simulink model "set_point_discreto"  (R2023b)
settings: Solver=VariableStepAuto  StartTime=0.0  StopTime=10.0  RelTol=1e-3
values from neighbouring files (symbols this model uses):
  r = 120.0    (= 120)    [controlador_foc_simulink.m]    (also in parametros_planta.m; params_subsistema_mecanico.m; sistema_completo_en_codigo.m)
  Ts = interp_ts(Ts_ts,t)    [calcular_metricas_operacion.m]
settings Model: Creator=Pc  LastModifiedBy=Pc

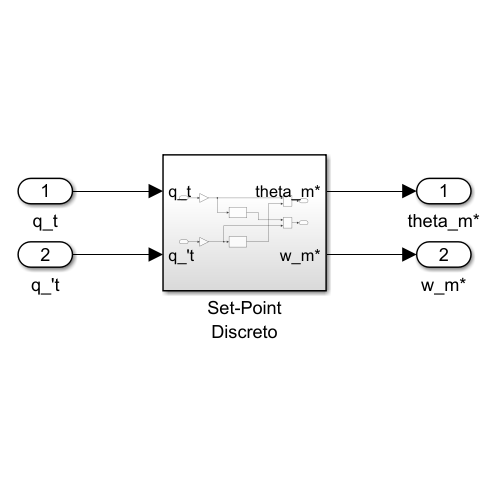
[thumbnail: Simulink's stored preview of the top-level diagram]
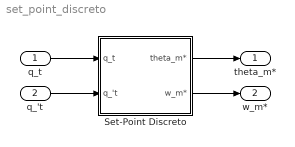
== system set_point_discreto ==
  q_t : Inport
  q_'t : Inport  Port=2
  Set-Point Discreto : Subsystem
  theta_m* : Outport
  w_m* : Outport  Port=2
  wires:
  Set-Point Discreto/1(theta_m*) -> theta_m*/1
  Set-Point Discreto/2(w_m*) -> w_m*/1
  q_t/1 -> Set-Point Discreto/1(q_t)
  q_'t/1 -> Set-Point Discreto/2(q_'t)

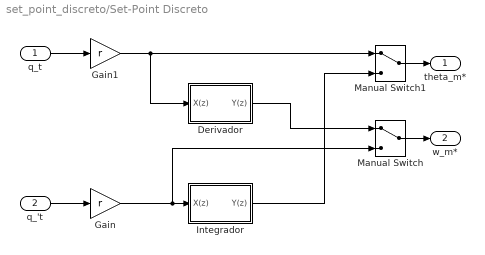
== system set_point_discreto/Set-Point Discreto ==
  q_t : Inport
  q_'t : Inport  Port=2
  "Derivador " : Subsystem
  Gain : Gain  Gain=r
  Gain1 : Gain  Gain=r
  Integrador : Subsystem
  Manual Switch : ManualSwitch
  Manual Switch1 : ManualSwitch
  theta_m* : Outport
  w_m* : Outport  Port=2
  wires:
  "Derivador "/1(Y(z)) -> Manual Switch/1
  Manual Switch/1 -> w_m*/1
  q_t/1 -> Gain1/1
  Gain1/1 -> "Derivador "/1(X(z)), Manual Switch1/1
  q_'t/1 -> Gain/1
  Manual Switch1/1 -> theta_m*/1
  Gain/1 -> Manual Switch/2, Integrador/1(X(z))
  Integrador/1(Y(z)) -> Manual Switch1/2

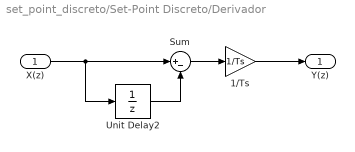
== system set_point_discreto/Set-Point Discreto/Derivador  ==
  X(z) : Inport
  1/Ts : Gain  Gain=1/Ts
  Sum : Sum  Inputs=|+-
  Unit Delay2 : UnitDelay  SampleTime=Ts  HasFrameUpgradeWarning=on
  Y(z) : Outport
  wires:
  Unit Delay2/1 -> Sum/2
  X(z)/1 -> Sum/1, Unit Delay2/1
  1/Ts/1 -> Y(z)/1
  Sum/1 -> 1/Ts/1

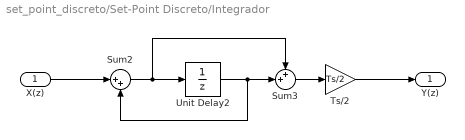
== system set_point_discreto/Set-Point Discreto/Integrador ==
  X(z) : Inport
  Sum2 : Sum  Inputs=|++
  Sum3 : Sum  Inputs=++|
  Ts/2 : Gain  Gain=Ts/2
  Unit Delay2 : UnitDelay  SampleTime=-1  HasFrameUpgradeWarning=on
  Y(z) : Outport
  wires:
  Ts/2/1 -> Y(z)/1
  Sum2/1 -> Unit Delay2/1, Sum3/1
  Sum3/1 -> Ts/2/1
  Unit Delay2/1 -> Sum2/2, Sum3/2
  X(z)/1 -> Sum2/1
